simulink model "dc_openloop_with_traj"  (R2020b)
settings: Solver=ode45  StartTime=0.0  StopTime=0.6  FixedStep=1e-6  RelTol=1e-6  AbsTol=1e-6
values from neighbouring files (symbols this model uses):
  c1 = 3*wmax/(t1*t1)    (= 349065.850399)    [dc_openloop_with_traj_data.m]
  c2 = -2*wmax/(t1*t1*t1)    (= -7757018.89775)    [dc_openloop_with_traj_data.m]
  d1 = c1    (= 349065.850399)    [dc_openloop_with_traj_data.m]
  d2 = c2    (= -7757018.89775)    [dc_openloop_with_traj_data.m]
  f = 0.4e-3    (= 0.0004)    [dc_openloop_with_traj_data.m]
  integrator_saturation = 10000    [dc_openloop_with_traj_data.m]
  J = 6e-5    (= 6e-05)    [dc_openloop_with_traj_data.m]
  Kb = 0.07    [dc_openloop_with_traj_data.m]
  KT = Kb    (= 0.07)    [dc_openloop_with_traj_data.m]
  L = 0.002    [dc_openloop_with_traj_data.m]
  R = 2    [dc_openloop_with_traj_data.m]
  t1 = 0.03    [dc_openloop_with_traj_data.m]
  t2 = t1+tc    (= 0.04)    [dc_openloop_with_traj_data.m]
  t3 = t2+t1    (= 0.07)    [dc_openloop_with_traj_data.m]
  tdd = 0*0.1    (= 0)    [dc_openloop_with_traj_data.m]
  vmax = 40    [dc_openloop_with_traj_data.m]
  wmax = thetaf/t1    (= 104.71975512)    [dc_openloop_with_traj_data.m]
libraries: simulink x7
settings Model: ExtModeTrigMode=oneshot  ExtModeArmWhenConnect=off  Creator=johnchiasson  LastModifiedBy=johnchiasson
settings SolverCC: AutoScaleAbsTol=off
settings DataIOCC: SaveFormat=Array  SignalLoggingSaveFormat=ModelDataLogs  SaveOutput=off  SaveTime=off  ReturnWorkspaceOutputs=off  SignalLoggingName=sigsOut
settings OptimizationCC: BlockReduction=off  BooleanDataType=off  ExpressionDepthLimit=2147483647  LifeSpan=inf
settings DebuggingCC: SaveWithParameterizedLinksMsg=none  UnderspecifiedInitializationDetection=Classic  MergeDetectMultiDrivingBlocksExec=none  SignalResolutionControl=TryResolveAllWithWarning  MultiTaskDSMMsg=warning  MultiTaskCondExecSysMsg=none  FcnCallInpInsideContextMsg=warning  StateNameClashWarn=warning  SFUnexpectedBacktrackingDiag=warning  SFNoUnconditionalDefaultTransitionDiag=warning  SFExecutionAtInitializationDiag=none  ArithmeticOperatorsInVariantConditions=warning
settings HardwareCC: ProdBitPerPointer=32  ProdBitPerSizeT=32  ProdBitPerPtrDiffT=32  ProdLargestAtomicFloat=None  ProdIntDivRoundTo=Undefined  ProdEndianess=Unspecified  ProdWordSize=32  ProdHWDeviceType=32-bit Generic  TargetUnknown=on
settings ModelReferenceCC: PropagateSignalLabelsOutOfModel=off
settings SFSimCC: SimUseLocalCustomCode=off  CustomCodeUndefinedFunction=UseInterfaceOnly
settings RTWCC: RTWUseLocalCustomCode=off
settings CodeAppCC: StateflowObjectComments=on
settings GRTTargetCC: TargetLangStandard=C89/C90 (ANSI)  CombineOutputUpdateFcns=off  GRTInterface=on
settings ConfigComp: CovMetricSettings=dw  CovSaveCumulativeToWorkspaceVar=on  CovSaveSingleToWorkspaceVar=on  CovExternalEMLEnable=off

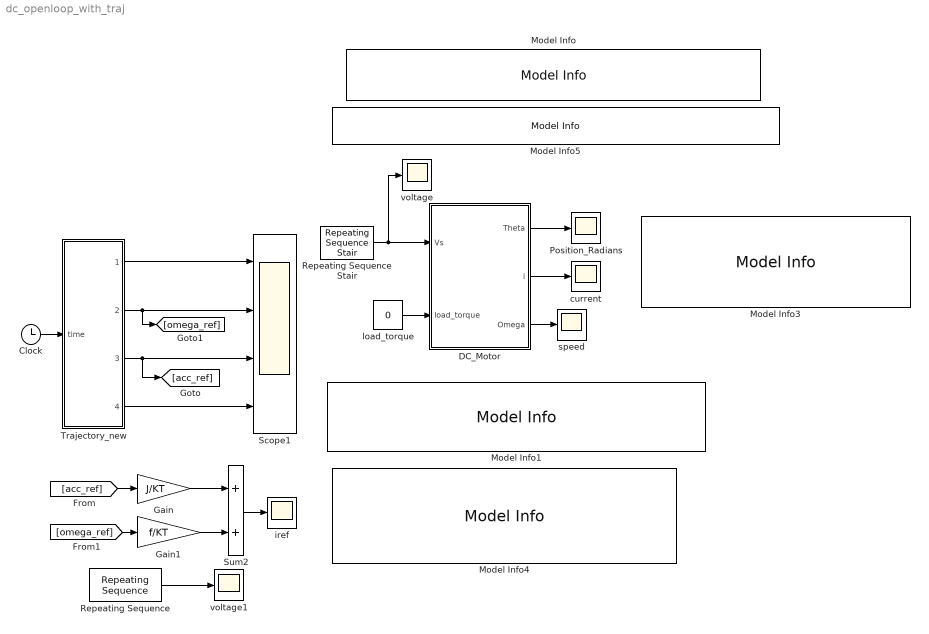
== system dc_openloop_with_traj ==
  Clock : Clock
  DC_Motor : Subsystem
  Gain : Gain  Gain=J/KT  SaturateOnIntegerOverflow=on  OutDataTypeStr=Inherit: Same as input  ParamDataTypeStr=Inherit: Same as input
  Gain1 : Gain  Gain=f/KT  SaturateOnIntegerOverflow=on  OutDataTypeStr=Inherit: Same as input  ParamDataTypeStr=Inherit: Same as input
  Model Info : simulink/Model-Wide Utilities/Model Info  Frame=on  DisplayStringWithTags=DC Servo Simulation Model  HorizontalTextAlignment=Center  LeftAlignmentValue=0.5
  Model Info1 : simulink/Model-Wide Utilities/Model Info  Frame=on  DisplayStringWithTags=COMMENTS Put your comments here to document your changes to the model  HorizontalTextAlignment=Left  LeftAlignmentValue=0.02
  Model Info3 : simulink/Model-Wide Utilities/Model Info  Frame=on  DisplayStringWithTags=|  HorizontalTextAlignment=Left  LeftAlignmentValue=0.02
      | SCOPE DATA
      | Open the scope block, select "parameters", 
      | then select  "data history" and 
      | UNCHECK  "Limit to last 5000 points" 
      | so you can save all your data.
  Model Info4 : simulink/Model-Wide Utilities/Model Info  Frame=on  DisplayStringWithTags=|  HorizontalTextAlignment=Left  LeftAlignmentValue=0.02
      | GOTO and FROM Blocks
      | Use these blocks so that the connecting lines do not cross.
      | 
      | Use the same background color for all "Goto" and 
      | "From" blocks of the SAME variable as illustrated.
  Model Info5 : simulink/Model-Wide Utilities/Model Info  Frame=on  DisplayStringWithTags=The integration algorithm is a variable step ODE45 with a tolerance of 1e-6  HorizontalTextAlignment=Left  LeftAlignmentValue=0.02
  Position_Radians : Scope
  Repeating Sequence : simulink/Sources/Repeating Sequence  rep_seq_t=[0 0.1 0.101 .2 0.201 0.3 0.301 0.4]  rep_seq_y=[10 10 0 0 -10 -10 0 0]
  Repeating Sequence Stair : simulink/Sources/Repeating Sequence Stair  OutValues=[10 0 -10 0 ]  tsamp=0.1  OutMin=[]  OutMax=[]  OutDataTypeStr=double  OutputDataTypeScalingMode=double  OutDataType=fixdt(0,8)  ConRadixGroup=Best Precision: Vector-wise  OutScaling=2^-12
  Scope1 : Scope  NumInputPorts=4
  Sum2 : Sum  InputSameDT=on  SaturateOnIntegerOverflow=on  OutDataTypeStr=Inherit: Same as first input
  Trajectory_new : Subsystem
  current : Scope
  iref : Scope
  load_torque : Constant  Value=0
  speed : Scope
  voltage : Scope
  voltage1 : Scope
  wires:
  Repeating Sequence Stair/1 -> DC_Motor/1(Vs), voltage/1
  DC_Motor/2(i) -> current/1
  load_torque/1 -> DC_Motor/2(load_torque)
  Clock/1 -> Trajectory_new/1(time)
  Trajectory_new/4(jerk_ref) -> Scope1/4
  Trajectory_new/3(alpha_ref) -> Scope1/3, [acc_ref]
  Trajectory_new/2(omega_ref) -> Scope1/2, [omega_ref]
  Trajectory_new/1(theta_ref) -> Scope1/1
  Gain/1 -> Sum2/1
  Gain1/1 -> Sum2/2
  [acc_ref] -> Gain/1
  [omega_ref] -> Gain1/1
  Sum2/1 -> iref/1
  DC_Motor/1(Theta) -> Position_Radians/1
  DC_Motor/3(Omega) -> speed/1
  Repeating Sequence/1 -> voltage1/1

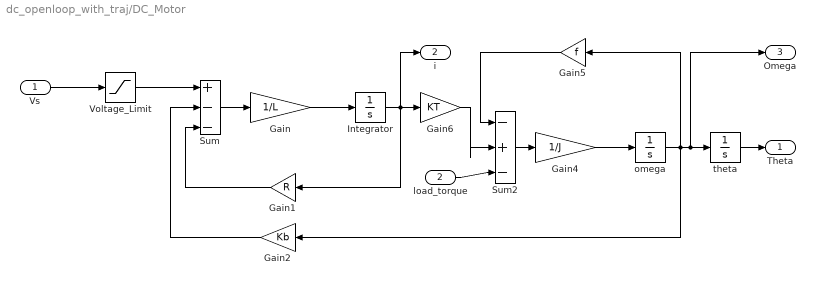
== system dc_openloop_with_traj/DC_Motor ==
  Vs : Inport
  load_torque : Inport  Port=2
  Gain : Gain  Gain=1/L  SaturateOnIntegerOverflow=on  OutDataTypeStr=Inherit: Same as input  ParamDataTypeStr=Inherit: Same as input
  Gain1 : Gain  Gain=R  SaturateOnIntegerOverflow=on  OutDataTypeStr=Inherit: Same as input  ParamDataTypeStr=Inherit: Same as input
  Gain2 : Gain  Gain=Kb  SaturateOnIntegerOverflow=on  OutDataTypeStr=Inherit: Same as input  ParamDataTypeStr=Inherit: Same as input
  Gain4 : Gain  Gain=1/J  SaturateOnIntegerOverflow=on  OutDataTypeStr=Inherit: Same as input  ParamDataTypeStr=Inherit: Same as input
  Gain5 : Gain  Gain=f  SaturateOnIntegerOverflow=on  OutDataTypeStr=Inherit: Same as input  ParamDataTypeStr=Inherit: Same as input
  Gain6 : Gain  Gain=KT  SaturateOnIntegerOverflow=on  OutDataTypeStr=Inherit: Same as input  ParamDataTypeStr=Inherit: Same as input
  Integrator : Integrator  UpperSaturationLimit=integrator_saturation  LowerSaturationLimit=-integrator_saturation
  Sum : Sum  Inputs=+--  InputSameDT=on  SaturateOnIntegerOverflow=on  OutDataTypeStr=Inherit: Same as first input
  Sum2 : Sum  Inputs=|-+-  InputSameDT=on  SaturateOnIntegerOverflow=on  OutDataTypeStr=Inherit: Same as first input
  Voltage_Limit : Saturate  UpperLimit=vmax  LowerLimit=-vmax
  omega : Integrator  UpperSaturationLimit=integrator_saturation  LowerSaturationLimit=-integrator_saturation
  theta : Integrator  UpperSaturationLimit=integrator_saturation  LowerSaturationLimit=-integrator_saturation
  Theta : Outport
  i : Outport  Port=2
  Omega : Outport  Port=3
  wires:
  Gain/1 -> Integrator/1
  Gain1/1 -> Sum/3
  Sum/1 -> Gain/1
  Vs/1 -> Voltage_Limit/1
  Integrator/1 -> Gain1/1, Gain6/1, i/1
  Sum2/1 -> Gain4/1
  Gain6/1 -> Sum2/2
  Gain4/1 -> omega/1
  load_torque/1 -> Sum2/3
  omega/1 -> Gain5/1, theta/1, Omega/1, Gain2/1
  Gain5/1 -> Sum2/1
  theta/1 -> Theta/1
  Gain2/1 -> Sum/2
  Voltage_Limit/1 -> Sum/1

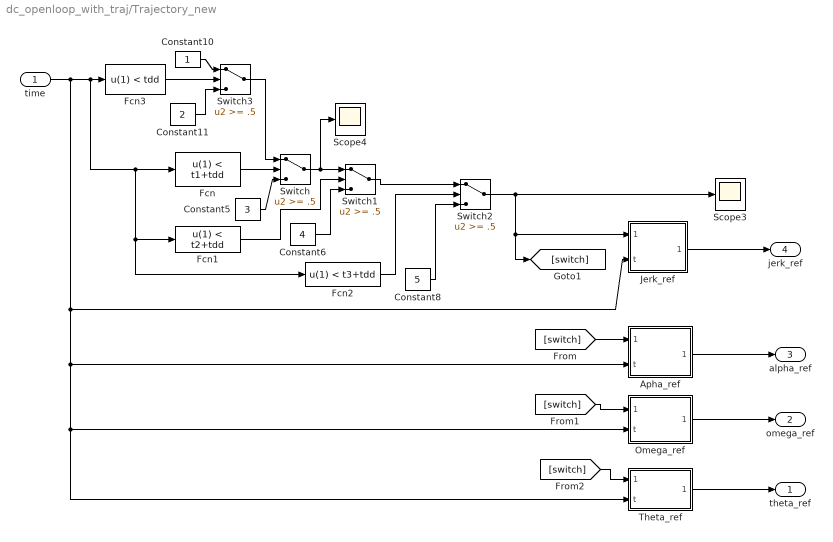
== system dc_openloop_with_traj/Trajectory_new ==
  time : Inport
  Apha_ref : Subsystem
  Constant10 : Constant
  Constant11 : Constant  Value=2
  Constant5 : Constant  Value=3
  Constant6 : Constant  Value=4
  Constant8 : Constant  Value=5
  Fcn : Fcn  Expr=u(1) < t1+tdd
  Fcn1 : Fcn  Expr=u(1) < t2+tdd
  Fcn2 : Fcn  Expr=u(1) < t3+tdd
  Fcn3 : Fcn  Expr=u(1) < tdd
  Jerk_ref : Subsystem
  Omega_ref : Subsystem
  Scope3 : Scope
  Scope4 : Scope
  Switch{,1..3} (4 alike) : Switch  Threshold=.5  SaturateOnIntegerOverflow=on  InputSameDT=on
  Theta_ref : Subsystem
  theta_ref : Outport
  omega_ref : Outport  Port=2
  alpha_ref : Outport  Port=3
  jerk_ref : Outport  Port=4
  wires:
  Fcn/1 -> Switch/2
  Constant5/1 -> Switch/3
  Constant6/1 -> Switch1/3
  Fcn1/1 -> Switch1/2
  Switch/1 -> Switch1/1, Scope4/1
  Fcn2/1 -> Switch2/2
  Constant8/1 -> Switch2/3
  Switch1/1 -> Switch2/1
  Switch3/1 -> Switch/1
  Constant10/1 -> Switch3/1
  Constant11/1 -> Switch3/3
  Fcn3/1 -> Switch3/2
  time/1 -> Fcn3/1, Fcn/1, Fcn1/1, Fcn2/1, Omega_ref/2(t), Theta_ref/2(t), Apha_ref/2(t), Jerk_ref/2(t)
  Jerk_ref/1(jerk_ref) -> jerk_ref/1
  Apha_ref/1(alpha_ref) -> alpha_ref/1
  Omega_ref/1(omega_ref) -> omega_ref/1
  Theta_ref/1(theta_ref) -> theta_ref/1
  Switch2/1 -> Scope3/1, Jerk_ref/1(switch), [switch]
  [switch] -> Apha_ref/1(switch)
  [switch] -> Omega_ref/1(switch)
  [switch] -> Theta_ref/1(switch)

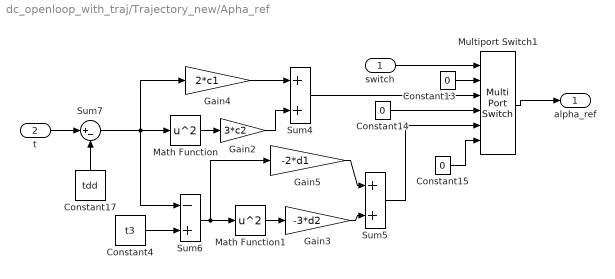
== system dc_openloop_with_traj/Trajectory_new/Apha_ref ==
  switch : Inport
  t : Inport  Port=2
  Constant13 : Constant  Value=0
  Constant14 : Constant  Value=0
  Constant15 : Constant  Value=0
  Constant17 : Constant  Value=tdd
  Constant4 : Constant  Value=t3
  Gain2 : Gain  Gain=3*c2  SaturateOnIntegerOverflow=on  OutDataTypeStr=Inherit: Same as input  ParamDataTypeStr=Inherit: Same as input
  Gain3 : Gain  Gain=-3*d2  SaturateOnIntegerOverflow=on  OutDataTypeStr=Inherit: Same as input  ParamDataTypeStr=Inherit: Same as input
  Gain4 : Gain  Gain=2*c1  SaturateOnIntegerOverflow=on  OutDataTypeStr=Inherit: Same as input  ParamDataTypeStr=Inherit: Same as input
  Gain5 : Gain  Gain=-2*d1  SaturateOnIntegerOverflow=on  OutDataTypeStr=Inherit: Same as input  ParamDataTypeStr=Inherit: Same as input
  Math Function : Math  Operator=square  SignedPower=on  SaturateOnIntegerOverflow=on
  Math Function1 : Math  Operator=square  SignedPower=on  SaturateOnIntegerOverflow=on
  Multiport Switch1 : MultiPortSwitch  Inputs=5  SaturateOnIntegerOverflow=on  InputSameDT=on
  Sum4 : Sum  Inputs=|++  InputSameDT=on  SaturateOnIntegerOverflow=on  OutDataTypeStr=Inherit: Same as first input
  Sum5 : Sum  Inputs=|++  InputSameDT=on  SaturateOnIntegerOverflow=on  OutDataTypeStr=Inherit: Same as first input
  Sum6 : Sum  Inputs=-+  InputSameDT=on  SaturateOnIntegerOverflow=on  OutDataTypeStr=Inherit: Same as first input
  Sum7 : Sum  Inputs=|+-  InputSameDT=on  SaturateOnIntegerOverflow=on  OutDataTypeStr=Inherit: Same as first input
  alpha_ref : Outport
  wires:
  t/1 -> Sum7/1
  Gain4/1 -> Sum4/1
  Gain2/1 -> Sum4/2
  Constant4/1 -> Sum6/2
  Gain5/1 -> Sum5/1
  Gain3/1 -> Sum5/2
  Sum5/1 -> Multiport Switch1/5
  Sum4/1 -> Multiport Switch1/3
  Constant14/1 -> Multiport Switch1/4
  Constant15/1 -> Multiport Switch1/6
  Constant13/1 -> Multiport Switch1/2
  Math Function/1 -> Gain2/1
  Math Function1/1 -> Gain3/1
  Sum6/1 -> Math Function1/1, Gain5/1
  Multiport Switch1/1 -> alpha_ref/1
  switch/1 -> Multiport Switch1/1
  Constant17/1 -> Sum7/2
  Sum7/1 -> Sum6/1, Gain4/1, Math Function/1

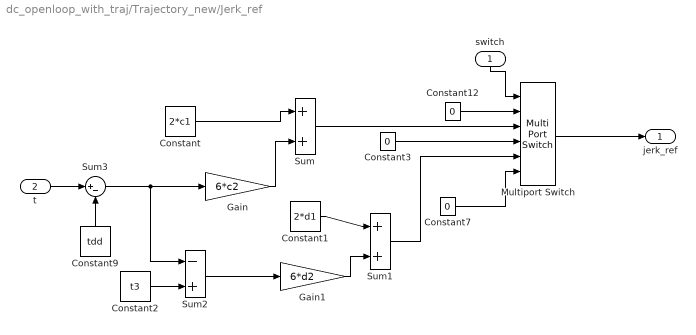
== system dc_openloop_with_traj/Trajectory_new/Jerk_ref ==
  switch : Inport
  t : Inport  Port=2
  Constant : Constant  Value=2*c1
  Constant1 : Constant  Value=2*d1
  Constant12 : Constant  Value=0
  Constant2 : Constant  Value=t3
  Constant3 : Constant  Value=0
  Constant7 : Constant  Value=0
  Constant9 : Constant  Value=tdd
  Gain : Gain  Gain=6*c2  SaturateOnIntegerOverflow=on  OutDataTypeStr=Inherit: Same as input  ParamDataTypeStr=Inherit: Same as input
  Gain1 : Gain  Gain=6*d2  SaturateOnIntegerOverflow=on  OutDataTypeStr=Inherit: Same as input  ParamDataTypeStr=Inherit: Same as input
  Multiport Switch : MultiPortSwitch  Inputs=5  SaturateOnIntegerOverflow=on  InputSameDT=on
  Sum : Sum  Inputs=|++  InputSameDT=on  SaturateOnIntegerOverflow=on  OutDataTypeStr=Inherit: Same as first input
  Sum1 : Sum  Inputs=|++  InputSameDT=on  SaturateOnIntegerOverflow=on  OutDataTypeStr=Inherit: Same as first input
  Sum2 : Sum  Inputs=-+  InputSameDT=on  SaturateOnIntegerOverflow=on  OutDataTypeStr=Inherit: Same as first input
  Sum3 : Sum  Inputs=|+-  InputSameDT=on  SaturateOnIntegerOverflow=on  OutDataTypeStr=Inherit: Same as first input
  jerk_ref : Outport
  wires:
  switch/1 -> Multiport Switch/1
  Constant/1 -> Sum/1
  Gain/1 -> Sum/2
  Constant2/1 -> Sum2/2
  Sum2/1 -> Gain1/1
  Constant1/1 -> Sum1/1
  Gain1/1 -> Sum1/2
  Sum1/1 -> Multiport Switch/5
  Sum/1 -> Multiport Switch/3
  Constant3/1 -> Multiport Switch/4
  Constant7/1 -> Multiport Switch/6
  Constant12/1 -> Multiport Switch/2
  Constant9/1 -> Sum3/2
  Sum3/1 -> Gain/1, Sum2/1
  Multiport Switch/1 -> jerk_ref/1
  t/1 -> Sum3/1

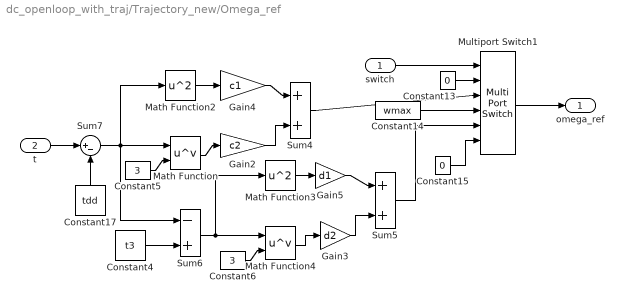
== system dc_openloop_with_traj/Trajectory_new/Omega_ref ==
  switch : Inport
  t : Inport  Port=2
  Constant13 : Constant  Value=0
  Constant14 : Constant  Value=wmax
  Constant15 : Constant  Value=0
  Constant17 : Constant  Value=tdd
  Constant4 : Constant  Value=t3
  Constant5 : Constant  Value=3
  Constant6 : Constant  Value=3
  Gain2 : Gain  Gain=c2  SaturateOnIntegerOverflow=on  OutDataTypeStr=Inherit: Same as input  ParamDataTypeStr=Inherit: Same as input
  Gain3 : Gain  Gain=d2  SaturateOnIntegerOverflow=on  OutDataTypeStr=Inherit: Same as input  ParamDataTypeStr=Inherit: Same as input
  Gain4 : Gain  Gain=c1  SaturateOnIntegerOverflow=on  OutDataTypeStr=Inherit: Same as input  ParamDataTypeStr=Inherit: Same as input
  Gain5 : Gain  Gain=d1  SaturateOnIntegerOverflow=on  OutDataTypeStr=Inherit: Same as input  ParamDataTypeStr=Inherit: Same as input
  Math Function : Math  Operator=pow  SignedPower=on  SaturateOnIntegerOverflow=on
  Math Function2 : Math  Operator=square  SignedPower=on  SaturateOnIntegerOverflow=on
  Math Function3 : Math  Operator=square  SignedPower=on  SaturateOnIntegerOverflow=on
  Math Function4 : Math  Operator=pow  SignedPower=on  SaturateOnIntegerOverflow=on
  Multiport Switch1 : MultiPortSwitch  Inputs=5  SaturateOnIntegerOverflow=on  InputSameDT=on
  Sum4 : Sum  Inputs=|++  InputSameDT=on  SaturateOnIntegerOverflow=on  OutDataTypeStr=Inherit: Same as first input
  Sum5 : Sum  Inputs=|++  InputSameDT=on  SaturateOnIntegerOverflow=on  OutDataTypeStr=Inherit: Same as first input
  Sum6 : Sum  Inputs=-+  InputSameDT=on  SaturateOnIntegerOverflow=on  OutDataTypeStr=Inherit: Same as first input
  Sum7 : Sum  Inputs=|+-  InputSameDT=on  SaturateOnIntegerOverflow=on  OutDataTypeStr=Inherit: Same as first input
  omega_ref : Outport
  wires:
  t/1 -> Sum7/1
  Gain4/1 -> Sum4/1
  Gain2/1 -> Sum4/2
  Constant4/1 -> Sum6/2
  Gain5/1 -> Sum5/1
  Gain3/1 -> Sum5/2
  Sum5/1 -> Multiport Switch1/5
  Sum4/1 -> Multiport Switch1/3
  Constant14/1 -> Multiport Switch1/4
  Constant15/1 -> Multiport Switch1/6
  Constant13/1 -> Multiport Switch1/2
  Math Function/1 -> Gain2/1
  Multiport Switch1/1 -> omega_ref/1
  switch/1 -> Multiport Switch1/1
  Constant17/1 -> Sum7/2
  Math Function2/1 -> Gain4/1
  Sum7/1 -> Sum6/1, Math Function/1, Math Function2/1
  Constant5/1 -> Math Function/2
  Math Function3/1 -> Gain5/1
  Sum6/1 -> Math Function4/1, Math Function3/1
  Constant6/1 -> Math Function4/2
  Math Function4/1 -> Gain3/1

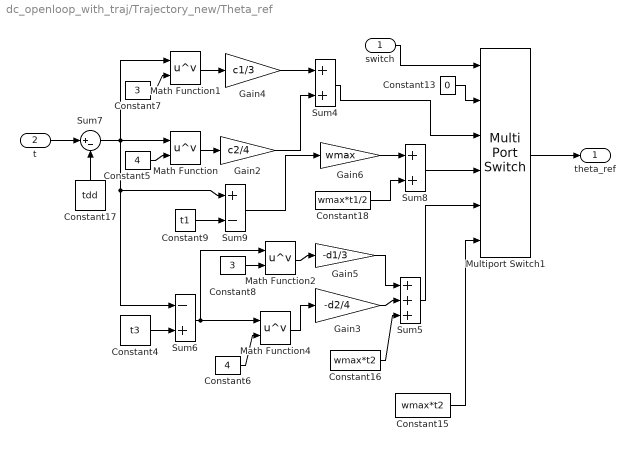
== system dc_openloop_with_traj/Trajectory_new/Theta_ref ==
  switch : Inport
  t : Inport  Port=2
  Constant13 : Constant  Value=0
  Constant15 : Constant  Value=wmax*t2
  Constant16 : Constant  Value=wmax*t2
  Constant17 : Constant  Value=tdd
  Constant18 : Constant  Value=wmax*t1/2
  Constant4 : Constant  Value=t3
  Constant5 : Constant  Value=4
  Constant6 : Constant  Value=4
  Constant7 : Constant  Value=3
  Constant8 : Constant  Value=3
  Constant9 : Constant  Value=t1
  Gain2 : Gain  Gain=c2/4  SaturateOnIntegerOverflow=on  OutDataTypeStr=Inherit: Same as input  ParamDataTypeStr=Inherit: Same as input
  Gain3 : Gain  Gain=-d2/4  SaturateOnIntegerOverflow=on  OutDataTypeStr=Inherit: Same as input  ParamDataTypeStr=Inherit: Same as input
  Gain4 : Gain  Gain=c1/3  SaturateOnIntegerOverflow=on  OutDataTypeStr=Inherit: Same as input  ParamDataTypeStr=Inherit: Same as input
  Gain5 : Gain  Gain=-d1/3  SaturateOnIntegerOverflow=on  OutDataTypeStr=Inherit: Same as input  ParamDataTypeStr=Inherit: Same as input
  Gain6 : Gain  Gain=wmax  SaturateOnIntegerOverflow=on  OutDataTypeStr=Inherit: Same as input  ParamDataTypeStr=Inherit: Same as input
  Math Function{,1..2,4} (4 alike) : Math  Operator=pow  SignedPower=on  SaturateOnIntegerOverflow=on
  Multiport Switch1 : MultiPortSwitch  Inputs=5  SaturateOnIntegerOverflow=on  InputSameDT=on
  Sum4 : Sum  InputSameDT=on  SaturateOnIntegerOverflow=on  OutDataTypeStr=Inherit: Same as first input
  Sum5 : Sum  Inputs=+++  InputSameDT=on  SaturateOnIntegerOverflow=on  OutDataTypeStr=Inherit: Same as first input
  Sum6 : Sum  Inputs=-+  InputSameDT=on  SaturateOnIntegerOverflow=on  OutDataTypeStr=Inherit: Same as first input
  Sum7 : Sum  Inputs=|+-  InputSameDT=on  SaturateOnIntegerOverflow=on  OutDataTypeStr=Inherit: Same as first input
  Sum8 : Sum  InputSameDT=on  SaturateOnIntegerOverflow=on  OutDataTypeStr=Inherit: Same as first input
  Sum9 : Sum  Inputs=+-  InputSameDT=on  SaturateOnIntegerOverflow=on  OutDataTypeStr=Inherit: Same as first input
  theta_ref : Outport
  wires:
  t/1 -> Sum7/1
  Gain4/1 -> Sum4/1
  Gain2/1 -> Sum4/2
  Sum4/1 -> Multiport Switch1/3
  Constant13/1 -> Multiport Switch1/2
  Math Function/1 -> Gain2/1
  Multiport Switch1/1 -> theta_ref/1
  switch/1 -> Multiport Switch1/1
  Math Function1/1 -> Gain4/1
  Sum7/1 -> Math Function/1, Math Function1/1, Sum6/1, Sum9/1
  Constant5/1 -> Math Function/2
  Constant7/1 -> Math Function1/2
  Gain5/1 -> Sum5/1
  Constant15/1 -> Multiport Switch1/6
  Constant17/1 -> Sum7/2
  Constant4/1 -> Sum6/2
  Gain3/1 -> Sum5/2
  Constant6/1 -> Math Function4/2
  Math Function4/1 -> Gain3/1
  Sum5/1 -> Multiport Switch1/5
  Math Function2/1 -> Gain5/1
  Sum6/1 -> Math Function4/1, Math Function2/1
  Constant8/1 -> Math Function2/2
  Constant16/1 -> Sum5/3
  Gain6/1 -> Sum8/1
  Sum8/1 -> Multiport Switch1/4
  Constant18/1 -> Sum8/2
  Constant9/1 -> Sum9/2
  Sum9/1 -> Gain6/1
